simulink model "MagnetotorquersDynamics_part2"  (R2012b)
settings: Solver=ode1  StartTime=0.0  StopTime=2000  FixedStep=0.1  RelTol=1e-3
InitFcn:
  | clear all;close all;clc;warning off all;
  | 
  | a=1/sqrt(3);
  | 
  | Z=[-a a a -a; -a -a a a; a a a a];
  | 
  | pinvZ=pinv(Z);
  | 
  | 
  | % Simulation run parameters
  | Rate=34.3; DeltaT=1/Rate;
  | 
  | % Maneuver Parameters
  | roll=0; pitch=0; yaw=30; roll=roll*pi/180; pitch=pitch*pi/180; yaw=yaw*pi/180;
  | SlewTime=5; SACengage=0;
  | Re=6371.2e3;mu=398601.2e9; %earth radius and universal gravitation constant
  | 
  | %Spacecraft orbit
  | h=180e3; %orbit altitude in meters
  | R=Re+h; %orbit radius from center of earth
  | we=0.000072921158553; %earth's angular velocity rad/solar sec(Vallado)
  | wo=sqrt(mu/(Re+h)^3);
  | 
  | 
  | %Spacecraft Inertia conditions
  | Ix=119.1259; Iy=150.6615; Iz=106.0288;
  | Ixy=0; Iyz=0; Ixz=0;
  | Imo=[Ix Ixy Ixz;
  | Ixy Iy Iyz;
  | Ixz Iyz Iz]; %Moment of inertia matrix
  | Iinv=inv(Imo); %Moment of inertia inverse goes in dynamics block
  | 
  | %Spacecraft initial Euler state angles and rates
  | phio=4*pi/180;thetao=-4*pi/180;psio=4*pi/180; %Initial Euler Angles
  | phidoto=0.15*pi/180;thetadoto=0.15*pi/180;psidoto=0.15*pi/180; %Initial Euler Rates
  | alfinit=[phio thetao psio];
  | winit=[phidoto thetadoto psidoto];
  | 
  | %Calculation of initial quaternion (qo) and angular momentum (Ho)
  | s1=sin(phio/2);s2=sin(thetao/2);s3=sin(psio/2);c1=cos(phio/2);c2=cos(thetao/2);c3=cos(psio/2);
  | q1o=s1*c2*c3-c1*s2*s3;
  | q2o=c1*s2*c3+s1*c2*s3; %Wie pg. 321
  | q3o=c1*c2*s3-s1*s2*c3;
  | q4o=c1*c2*c3+s1*s2*s3;
  | S1=sin(phio);S2=sin(thetao);S3=sin(psio);C1=cos(phio);C2=cos(thetao);C3=cos(psio);
  | wxo=phidoto-psidoto*S2-wo*S3*C2;
  | wyo=thetadoto*C1+psidoto*C2*S1-wo*(C3*C1+S3*S2*S1);
  | wzo=psidoto*C2*C1-thetadoto*S1-wo*(S3*S2*C1-C3*S1);
  | qo=[q1o q2o q3o q4o];
  | Ho=Imo*[wxo wyo wzo]';
  | 
  | x=[4 4 4 2 2 2];%xmax
  | u=[2.1 2.1 2.1];%umax
  | J=[Ix Iy Iz];  % J of the system
  | 
  | Jinv=J';
  | 
  | hom=0.001; %rad/s
  | N=0;
  | %Linear quadratic Regulator
  | A=[0,0,0,1,0,0;0,0,0,0,1,0;0,0,0,0,0,1;4*((J(3)-J(2))/J(1))*(hom^2),0,0,0,0,((J(3)+J(1)-J(2))/J(1))*hom;0,3*((J(3)-J(1))/J(2))*(hom^2),0,0,0,0;0,0,((J(1)-J(2))/J(3))*(hom^2),(((J(2)-J(1)-J(3))/J(3))*hom),0,0];
  | B=[0,0,0;0,0,0;0,0,0;1/J(1),0,0;0,1/J(2),0;0,0,1/J(3)];
  | Q=[1/(x(1)^2),0,0,0,0,0;0,1/(x(2)^2),0,0,0,0;0,0,1/(x(3)^2),0,0,0;0,0,0,1/(x(4)^2),0,0;0,0,0,0,1/(x(5)^2),0;0,0,0,0,0,1/(x(6)^2)];
  | R=[100/(u(1)^2),0,0;0,100/(u(2)^2),0;0,0,100/(u(3)^2)];
  | 
  |  K=lqr(A,B,Q,R,N);
  | 
  | %State Estimator
  | 
  | %C=[1,0,0,0,0,0;0,1,0,0,0,0;0,0,1,0,0,0;0,0,0,0,0,0;0,0,0,0,0,0;0,0,0,0,0,0];
  | 
  | C=eye(6,6);
  | Q1=eye(6,6);
  | R1=eye(6,6);
  | 
  | L=[lqr(A',C',Q1,R1)]';
  | 
  | %Magnetic Field
  | 
  | Bxe=22791*10^(-9);% nT
  | Bye=0;
  | Bze=-11452*10^(-9);
  | 
  | Bx=22.791;% nT
  | By=0;
  | Bz=-11.452;
  | 
  | Be=[Bxe Bye Bze];
  | 
  | Bi=[Bx By Bz];
  | 
  | B=[0 Bz -By; -Bz 0 Bx; By -Bx 0];
  | 
  | Intialrate=[1.8*pi/180;1.8*pi/180;1.8*pi/180];
  | 
  | %Intialrate=[1.8*pi/180;0;1.8*pi/180];
  | %Intialrate=[0.8*pi/180;0.8*pi/180;0.8*pi/180];
  | 
  | BoB=1;
libraries: aerospace x7
settings Model: Creator=bleonard  LastModifiedBy=Grompone
settings DataIOCC: SignalLoggingSaveFormat=ModelDataLogs
settings OptimizationCC: InitFltsAndDblsToZero=on
settings DebuggingCC: SaveWithParameterizedLinksMsg=none  MultiTaskCondExecSysMsg=none  FcnCallInpInsideContextMsg=EnableAllAsWarning  StrictBusMsg=None
settings RTWCC: IncludeERTFirstTime=on
settings GRTTargetCC: CombineOutputUpdateFcns=off  GRTInterface=on

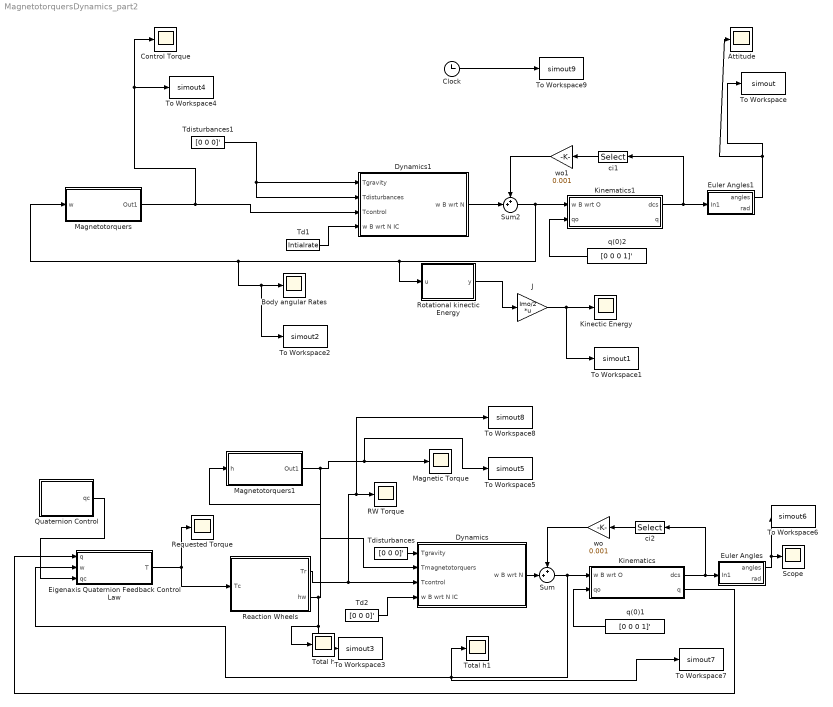
== system MagnetotorquersDynamics_part2 ==
  Attitude : Scope
      settings: YMin=-200  YMax=200  SaveName=ScopeData2
  Body angular Rates : Scope
      settings: YMin=-0.04  YMax=0.05  SaveName=ScopeData7
  Clock : Clock
  Control Torque : Scope
      settings: YMin=-1e-06  YMax=1.75e-06  SaveName=ScopeData5
  Dynamics : Subsystem
  Dynamics1 : Subsystem
  Eigenaxis Quaternion Feedback Control Law : Subsystem
  Euler Angles : Subsystem
  Euler Angles1 : Subsystem
  J : Gain  Gain=Imo/2  Multiplication=Matrix(K*u)  SaturateOnIntegerOverflow=on  OutDataTypeStr=Inherit: Same as input  ParamDataTypeStr=Inherit: Same as input
  Kinectic Energy : Scope
      settings: ShowLegends=on  YMin=-200  YMax=200  SaveName=ScopeData12
  Kinematics : Subsystem
  Kinematics1 : Subsystem
  Magnetic Torque : Scope
      settings: YMin=-7e-09  YMax=8e-09  SaveName=ScopeData15
  Magnetotorquers : Subsystem
  Magnetotorquers1 : Subsystem
  Quaternion Control : MATLAB Function  TreatAsAtomicUnit=on
  RW Torque : Scope
      settings: SaveName=ScopeData10
  Reaction Wheels : Subsystem
  Requested Torque : Scope
  Rotational kinectic Energy : MATLAB Function  TreatAsAtomicUnit=on
  Scope : Scope
      settings: YMin=-200  YMax=200
  Sum : Sum  Inputs=++|
  Sum2 : Sum  Inputs=++|
  Td1 : Constant  Value=Intialrate
  Td2 : Constant  Value=[0 0 0]'
  Tdisturbances : Constant  Value=[0 0 0]'
  Tdisturbances1 : Constant  Value=[0 0 0]'
  To Workspace : ToWorkspace  VariableName=simout  SampleTime=-1  SaveFormat=Timeseries
  To Workspace1 : ToWorkspace  VariableName=simout1  SampleTime=-1  SaveFormat=Timeseries
  To Workspace2 : ToWorkspace  VariableName=simout2  SampleTime=-1  SaveFormat=Timeseries
  To Workspace3 : ToWorkspace  VariableName=simout3  SampleTime=-1  SaveFormat=Timeseries
  To Workspace4 : ToWorkspace  VariableName=simout4  SampleTime=-1  SaveFormat=Timeseries
  To Workspace5 : ToWorkspace  VariableName=simout5  SampleTime=-1  SaveFormat=Timeseries
  To Workspace6 : ToWorkspace  VariableName=simout6  SampleTime=-1  SaveFormat=Timeseries
  To Workspace7 : ToWorkspace  VariableName=simout7  SampleTime=-1  SaveFormat=Timeseries
  To Workspace8 : ToWorkspace  VariableName=simout8  SampleTime=-1  SaveFormat=Timeseries
  To Workspace9 : ToWorkspace  VariableName=simout9  SampleTime=-1  SaveFormat=Timeseries
  Total h : Scope
      settings: YMin=-7e-09  YMax=8e-09  SaveName=ScopeData16
  Total h1 : Scope
      settings: YMin=-7e-09  YMax=8e-09  SaveName=ScopeData3
  ci1 : Selector  InputPortWidth=9  IndexOptions=Index vector (dialog)  Indices=[4 5 6]  OutputSizes=1
  ci2 : Selector  InputPortWidth=9  IndexOptions=Index vector (dialog)  Indices=[4 5 6]  OutputSizes=1
  q(0)1 : Constant  Value=[0 0 0 1]'
  q(0)2 : Constant  Value=[0 0 0 1]'
  wo : Gain  Gain=0.001
  wo1 : Gain  Gain=0.001
  wires:
  Sum/1 -> Total h1/1, To Workspace7/1, Eigenaxis Quaternion Feedback Control Law/2(w), Kinematics/1(w B wrt O)
  Kinematics/1(dcs) -> ci2/1, Euler Angles/1(In1)
  ci2/1 -> wo/1
  Euler Angles/1(angles) -> Scope/1, To Workspace6/1
  Kinematics/2(q) -> Eigenaxis Quaternion Feedback Control Law/1(q)
  Tdisturbances/1 -> Dynamics/1(Tgravity)
  Td2/1 -> Dynamics/4(w B wrt N IC)
  wo/1 -> Sum/1
  Eigenaxis Quaternion Feedback Control Law/1(T) -> Reaction Wheels/1(Tc), Requested Torque/1
  Reaction Wheels/1(Tr) -> To Workspace8/1, RW Torque/1, Dynamics/3(Tcontrol)
  Dynamics/1(w B wrt N) -> Sum/2
  q(0)1/1 -> Kinematics/2(qo)
  Quaternion Control/1(qc) -> Eigenaxis Quaternion Feedback Control Law/3(qc)
  Sum2/1 -> Rotational kinectic Energy/1(u), To Workspace2/1, Body angular Rates/1, Magnetotorquers/1(w), Kinematics1/1(w B wrt O)
  Kinematics1/1(dcs) -> ci1/1, Euler Angles1/1(In1)
  ci1/1 -> wo1/1
  Euler Angles1/1(angles) -> Attitude/1, To Workspace/1
  Tdisturbances1/1 -> Dynamics1/1(Tgravity), Dynamics1/2(Tdisturbances)
  Magnetotorquers/1(Out1) -> To Workspace4/1, Control Torque/1, Dynamics1/3(Tcontrol)
  Dynamics1/1(w B wrt N) -> Sum2/2
  q(0)2/1 -> Kinematics1/2(qo)
  Td1/1 -> Dynamics1/4(w B wrt N IC)
  wo1/1 -> Sum2/1
  Magnetotorquers1/1(Out1) -> Dynamics/2(Tmagnetotorquers), To Workspace5/1, Magnetic Torque/1
  Rotational kinectic Energy/1(y) -> J/1
  J/1 -> To Workspace1/1, Kinectic Energy/1
  Reaction Wheels/2(hw) -> Total h/1, To Workspace3/1, Magnetotorquers1/1(h)
  Clock/1 -> To Workspace9/1

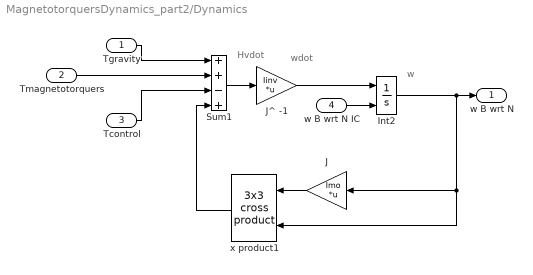
== system MagnetotorquersDynamics_part2/Dynamics ==
  note: wdot
  note: Hvdot
  note: w
  Tgravity : Inport
  Tmagnetotorquers : Inport  Port=2
  Tcontrol : Inport  Port=3
  w B wrt N IC : Inport  Port=4
  "   J^ -1" : Gain  Gain=Iinv  Multiplication=Matrix(K*u)  SaturateOnIntegerOverflow=on  OutDataTypeStr=Inherit: Same as input  ParamDataTypeStr=Inherit: Same as input
  Int2 : Integrator  InitialConditionSource=external  InitialCondition="[0  -0.001  0]'"
  J : Gain  Gain=Imo  Multiplication=Matrix(K*u)  SaturateOnIntegerOverflow=on  OutDataTypeStr=Inherit: Same as input  ParamDataTypeStr=Inherit: Same as input
  Sum1 : Sum  Inputs=++-+  SaturateOnIntegerOverflow=on  InputSameDT=on  OutDataTypeStr=Inherit: Same as first input
  x product1 : aerospace/Axes Transformations/3x3 cross product
  w B wrt N : Outport
  wires:
  Sum1/1 -> "   J^ -1"/1
  Int2/1 -> J/1, x product1/2, w B wrt N/1
  x product1/1 -> Sum1/4
  "   J^ -1"/1 -> Int2/1
  J/1 -> x product1/1
  Tgravity/1 -> Sum1/1
  Tmagnetotorquers/1 -> Sum1/2
  Tcontrol/1 -> Sum1/3
  w B wrt N IC/1 -> Int2/2

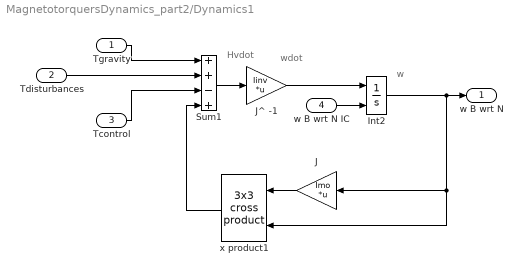
== system MagnetotorquersDynamics_part2/Dynamics1 ==
  note: wdot
  note: Hvdot
  note: w
  Tgravity : Inport
  Tdisturbances : Inport  Port=2
  Tcontrol : Inport  Port=3
  w B wrt N IC : Inport  Port=4
  "   J^ -1" : Gain  Gain=Iinv  Multiplication=Matrix(K*u)  SaturateOnIntegerOverflow=on  OutDataTypeStr=Inherit: Same as input  ParamDataTypeStr=Inherit: Same as input
  Int2 : Integrator  InitialConditionSource=external  InitialCondition="[0  -0.001  0]'"
  J : Gain  Gain=Imo  Multiplication=Matrix(K*u)  SaturateOnIntegerOverflow=on  OutDataTypeStr=Inherit: Same as input  ParamDataTypeStr=Inherit: Same as input
  Sum1 : Sum  Inputs=++-+  SaturateOnIntegerOverflow=on  InputSameDT=on  OutDataTypeStr=Inherit: Same as first input
  x product1 : aerospace/Axes Transformations/3x3 cross product
  w B wrt N : Outport
  wires:
  Sum1/1 -> "   J^ -1"/1
  Int2/1 -> J/1, x product1/2, w B wrt N/1
  x product1/1 -> Sum1/4
  "   J^ -1"/1 -> Int2/1
  J/1 -> x product1/1
  Tgravity/1 -> Sum1/1
  Tdisturbances/1 -> Sum1/2
  Tcontrol/1 -> Sum1/3
  w B wrt N IC/1 -> Int2/2

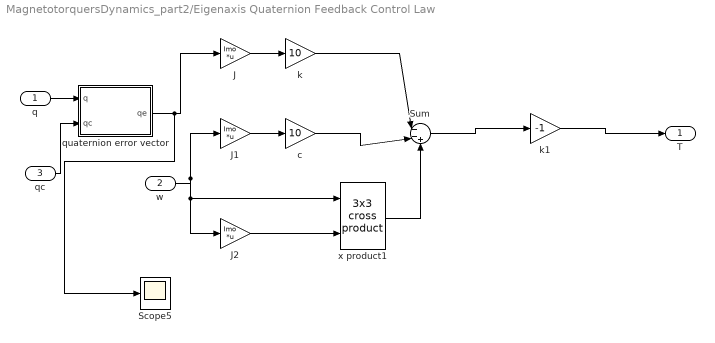
== system MagnetotorquersDynamics_part2/Eigenaxis Quaternion Feedback Control Law ==
  q : Inport
  w : Inport  Port=2
  qc : Inport  Port=3
  J : Gain  Gain=Imo  Multiplication=Matrix(K*u)
  J1 : Gain  Gain=Imo  Multiplication=Matrix(K*u)
  J2 : Gain  Gain=Imo  Multiplication=Matrix(K*u)
  Scope5 : Scope
      settings: YMin=-200  YMax=200  SaveName=ScopeData6
  Sum : Sum  Inputs=|--+
  c : Gain  Gain=10
  k : Gain  Gain=10
  k1 : Gain  Gain=-1
  quaternion error vector : MATLAB Function  TreatAsAtomicUnit=on
  x product1 : aerospace/Axes Transformations/3x3 cross product
  T : Outport
  wires:
  J/1 -> k/1
  quaternion error vector/1(qe) -> Scope5/1, J/1
  J1/1 -> c/1
  w/1 -> J1/1, x product1/1, J2/1
  k/1 -> Sum/1
  c/1 -> Sum/2
  x product1/1 -> Sum/3
  q/1 -> quaternion error vector/1(q)
  qc/1 -> quaternion error vector/2(qc)
  J2/1 -> x product1/2
  Sum/1 -> k1/1
  k1/1 -> T/1

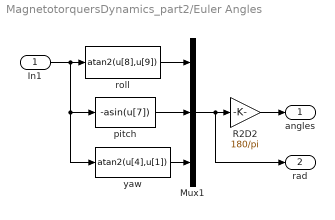
== system MagnetotorquersDynamics_part2/Euler Angles ==
  In1 : Inport
  Mux1 : Mux  Inputs=3
  R2D2 : Gain  Gain=180/pi  SampleTime=0.1
  pitch : Fcn  Expr=-asin(u[7])
  roll : Fcn  Expr=atan2(u[8],u[9])
  yaw : Fcn  Expr=atan2(u[4],u[1])
  angles : Outport
  rad : Outport  Port=2
  wires:
  roll/1 -> Mux1/1
  yaw/1 -> Mux1/3
  pitch/1 -> Mux1/2
  Mux1/1 -> rad/1, R2D2/1
  In1/1 -> roll/1, pitch/1, yaw/1
  R2D2/1 -> angles/1

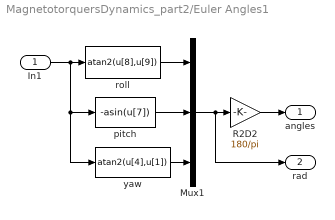
== system MagnetotorquersDynamics_part2/Euler Angles1 ==
  In1 : Inport
  Mux1 : Mux  Inputs=3
  R2D2 : Gain  Gain=180/pi  SampleTime=0.1
  pitch : Fcn  Expr=-asin(u[7])
  roll : Fcn  Expr=atan2(u[8],u[9])
  yaw : Fcn  Expr=atan2(u[4],u[1])
  angles : Outport
  rad : Outport  Port=2
  wires:
  roll/1 -> Mux1/1
  yaw/1 -> Mux1/3
  pitch/1 -> Mux1/2
  Mux1/1 -> rad/1, R2D2/1
  In1/1 -> roll/1, pitch/1, yaw/1
  R2D2/1 -> angles/1

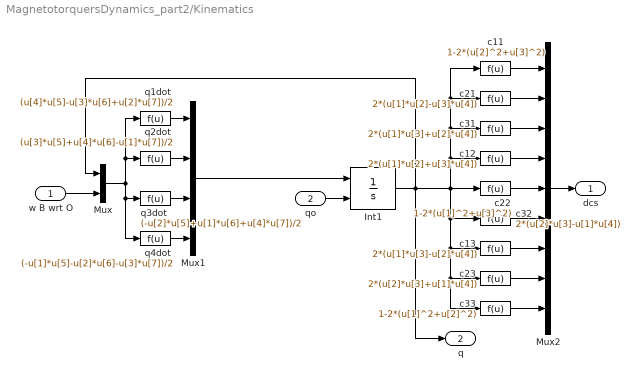
== system MagnetotorquersDynamics_part2/Kinematics ==
  w B wrt O : Inport
  qo : Inport  Port=2
  Int1 : Integrator  InitialConditionSource=external  InitialCondition=[0 0 -0.1]'
  Mux : Mux  Inputs=2
  Mux1 : Mux
  Mux2 : Mux  Inputs=9
  c11 : Fcn  Expr=1-2*(u[2]^2+u[3]^2)
  c12 : Fcn  Expr=2*(u[1]*u[2]+u[3]*u[4])
  c13 : Fcn  Expr=2*(u[1]*u[3]-u[2]*u[4])
  c21 : Fcn  Expr=2*(u[1]*u[2]-u[3]*u[4])
  c22 : Fcn  Expr=1-2*(u[1]^2+u[3]^2)
  c23 : Fcn  Expr=2*(u[2]*u[3]+u[1]*u[4])
  c31 : Fcn  Expr=2*(u[1]*u[3]+u[2]*u[4])
  c32 : Fcn  Expr=2*(u[2]*u[3]-u[1]*u[4])
  c33 : Fcn  Expr=1-2*(u[1]^2+u[2]^2)
  q1dot : Fcn  Expr=(u[4]*u[5]-u[3]*u[6]+u[2]*u[7])/2
  q2dot : Fcn  Expr=(u[3]*u[5]+u[4]*u[6]-u[1]*u[7])/2
  q3dot : Fcn  Expr=(-u[2]*u[5]+u[1]*u[6]+u[4]*u[7])/2
  q4dot : Fcn  Expr=(-u[1]*u[5]-u[2]*u[6]-u[3]*u[7])/2
  dcs : Outport
  q : Outport  Port=2
  wires:
  Mux/1 -> q4dot/1, q3dot/1, q1dot/1, q2dot/1
  q1dot/1 -> Mux1/1
  q2dot/1 -> Mux1/2
  q3dot/1 -> Mux1/3
  q4dot/1 -> Mux1/4
  Int1/1 -> Mux/1, c22/1, c11/1, c21/1, c31/1, c12/1, c32/1, c13/1, c33/1, c23/1, q/1
  c11/1 -> Mux2/1
  c22/1 -> Mux2/5
  c33/1 -> Mux2/9
  c21/1 -> Mux2/2
  c31/1 -> Mux2/3
  c12/1 -> Mux2/4
  c32/1 -> Mux2/6
  c13/1 -> Mux2/7
  c23/1 -> Mux2/8
  Mux1/1 -> Int1/1
  w B wrt O/1 -> Mux/2
  Mux2/1 -> dcs/1
  qo/1 -> Int1/2

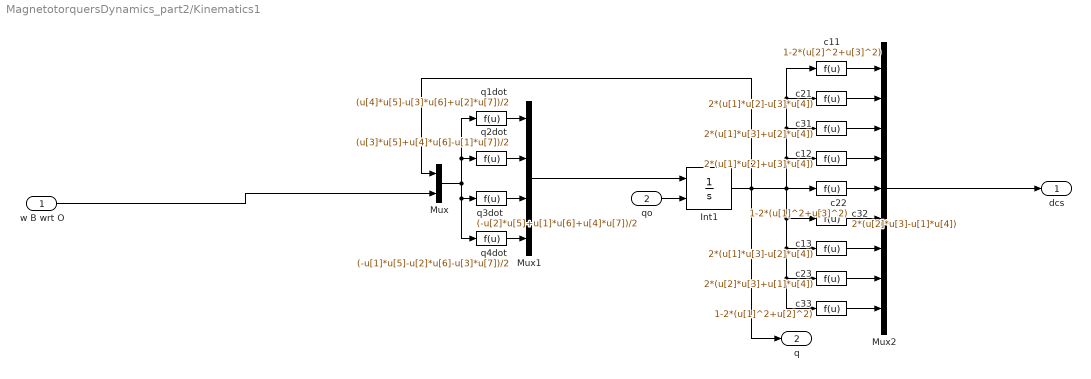
== system MagnetotorquersDynamics_part2/Kinematics1 ==
  w B wrt O : Inport
  qo : Inport  Port=2
  Int1 : Integrator  InitialConditionSource=external  InitialCondition=[0 0 -0.1]'
  Mux : Mux  Inputs=2
  Mux1 : Mux
  Mux2 : Mux  Inputs=9
  c11 : Fcn  Expr=1-2*(u[2]^2+u[3]^2)
  c12 : Fcn  Expr=2*(u[1]*u[2]+u[3]*u[4])
  c13 : Fcn  Expr=2*(u[1]*u[3]-u[2]*u[4])
  c21 : Fcn  Expr=2*(u[1]*u[2]-u[3]*u[4])
  c22 : Fcn  Expr=1-2*(u[1]^2+u[3]^2)
  c23 : Fcn  Expr=2*(u[2]*u[3]+u[1]*u[4])
  c31 : Fcn  Expr=2*(u[1]*u[3]+u[2]*u[4])
  c32 : Fcn  Expr=2*(u[2]*u[3]-u[1]*u[4])
  c33 : Fcn  Expr=1-2*(u[1]^2+u[2]^2)
  q1dot : Fcn  Expr=(u[4]*u[5]-u[3]*u[6]+u[2]*u[7])/2
  q2dot : Fcn  Expr=(u[3]*u[5]+u[4]*u[6]-u[1]*u[7])/2
  q3dot : Fcn  Expr=(-u[2]*u[5]+u[1]*u[6]+u[4]*u[7])/2
  q4dot : Fcn  Expr=(-u[1]*u[5]-u[2]*u[6]-u[3]*u[7])/2
  dcs : Outport
  q : Outport  Port=2
  wires:
  Mux/1 -> q4dot/1, q3dot/1, q1dot/1, q2dot/1
  q1dot/1 -> Mux1/1
  q2dot/1 -> Mux1/2
  q3dot/1 -> Mux1/3
  q4dot/1 -> Mux1/4
  Int1/1 -> Mux/1, c22/1, c11/1, c21/1, c31/1, c12/1, c32/1, c13/1, c33/1, c23/1, q/1
  c11/1 -> Mux2/1
  c22/1 -> Mux2/5
  c33/1 -> Mux2/9
  c21/1 -> Mux2/2
  c31/1 -> Mux2/3
  c12/1 -> Mux2/4
  c32/1 -> Mux2/6
  c13/1 -> Mux2/7
  c23/1 -> Mux2/8
  Mux1/1 -> Int1/1
  qo/1 -> Int1/2
  w B wrt O/1 -> Mux/2
  Mux2/1 -> dcs/1

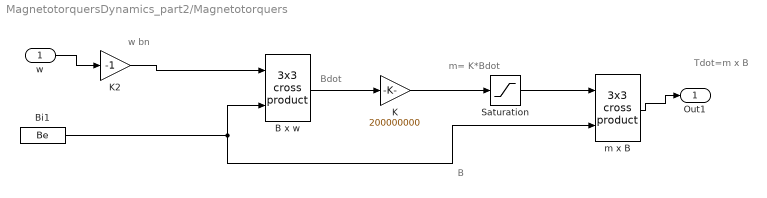
== system MagnetotorquersDynamics_part2/Magnetotorquers ==
  note: w bn
  note: B
  note: m= K*Bdot
  note: Tdot=m x B
  note: Bdot
  w : Inport
  B x w : aerospace/Axes Transformations/3x3 cross product
  Bi1 : Constant  Value=Be
  K : Gain  Gain=200000000
  K2 : Gain  Gain=-1
  Saturation : Saturate  UpperLimit=110  LowerLimit=-110
  m x B : aerospace/Axes Transformations/3x3 cross product
  Out1 : Outport
  wires:
  B x w/1 -> K/1
  m x B/1 -> Out1/1
  K/1 -> Saturation/1
  w/1 -> K2/1
  Bi1/1 -> m x B/2, B x w/2
  K2/1 -> B x w/1
  Saturation/1 -> m x B/1

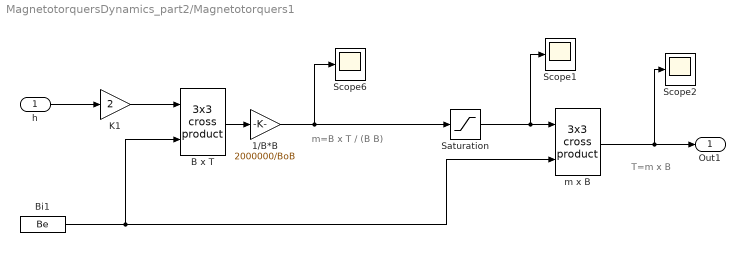
== system MagnetotorquersDynamics_part2/Magnetotorquers1 ==
  note: m=B x T / (B B)
  note: T=m x B
  h : Inport
  1/B*B : Gain  Gain=2000000/BoB
  B x T : aerospace/Axes Transformations/3x3 cross product
  Bi1 : Constant  Value=Be
  K1 : Gain  Gain=2
  Saturation : Saturate  UpperLimit=110  LowerLimit=-110
  Scope1 : Scope
      settings: YMin=-6.5  YMax=0.5  SaveName=ScopeData9
  Scope2 : Scope
      settings: YMin=-0.000225  YMax=0.00035  SaveName=ScopeData11
  Scope6 : Scope
      settings: YMin=-0.00225  YMax=0.002  SaveName=ScopeData8
  m x B : aerospace/Axes Transformations/3x3 cross product
  Out1 : Outport
  wires:
  m x B/1 -> Scope2/1, Out1/1
  Saturation/1 -> Scope1/1, m x B/1
  h/1 -> K1/1
  K1/1 -> B x T/1
  Bi1/1 -> m x B/2, B x T/2
  B x T/1 -> 1/B*B/1
  1/B*B/1 -> Scope6/1, Saturation/1

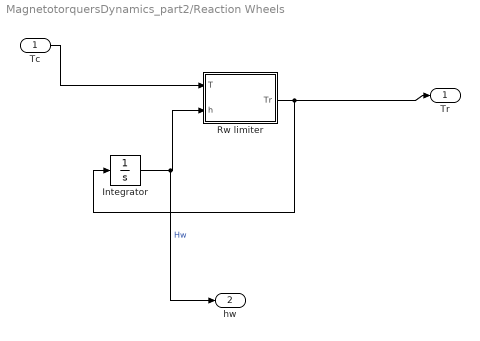
== system MagnetotorquersDynamics_part2/Reaction Wheels ==
  Tc : Inport
  Integrator : Integrator  InitialCondition=[0 0 0]
  Rw limiter : MATLAB Function  TreatAsAtomicUnit=on
  Tr : Outport
  hw : Outport  Port=2
  wires:
  Integrator/1 -> hw/1, Rw limiter/2(h)  "Hw"
  Rw limiter/1(Tr) -> Integrator/1, Tr/1
  Tc/1 -> Rw limiter/1(T)

== matlab function MagnetotorquersDynamics_part2/Quaternion Control ==
  data: qc output
function qc = fcn
%#codegen

alfa=120*pi/180;

e1=1/sqrt(3);
e2=1/sqrt(3);
e3=1/sqrt(3);


q1=sin(alfa/2)*e1;
q2=sin(alfa/2)*e2;
q3=sin(alfa/2)*e3;
q4=cos(alfa/2);


qc = [q1 q2 q3 q4];

== matlab function MagnetotorquersDynamics_part2/Reaction Wheels/Rw limiter ==
  data: T input; Tr output; h input
function Tr = fcn(T,h)
%#eml



hmax=20; %absolute maximum momentum RW

Tmax=0.1; %absolute maximum Torque RW

Trc=zeros(3,1);
Tr=zeros(3,1);

if abs(h(1))<hmax

if abs(T(1))>Tmax
    
    Trc(1)=Tmax;
    
else
    
    Trc(1)=abs(T(1));
    
end

else
    
  Trc(1)=0;
  
end

Tr(1)=sign(T(1))*Trc(1);

if abs(h(2))<hmax

if abs(T(2))>Tmax
    
    Trc(2)=Tmax;
    
else
    
    Trc(2)=abs(T(2));
    
end

else
    
  Trc(2)=0;
  
end

Tr(2)=sign(T(2))*Trc(2);

if abs(h(3))<hmax

if abs(T(3))>Tmax
    
    Trc(3)=Tmax;
    
else
    
    Trc(3)=abs(T(3));
    
end

else
    
  Trc(3)=0;
  
end

Tr(3)=sign(T(3))*Trc(3);

== matlab function MagnetotorquersDynamics_part2/Eigenaxis Quaternion Feedback Control Law/quaternion error vector ==
  data: q input; qe output; qc input
function qe = fcn(q,qc)
%#codegen

qcm=[qc(4) qc(3) -qc(2) -qc(1);-qc(3) qc(4) qc(1) -qc(2);qc(2) -qc(1) qc(4) -qc(3);qc(1) qc(2) qc(3) qc(4)];


qem = qcm*q; 

qe=[qem(1) qem(2) qem(3)]';

== matlab function MagnetotorquersDynamics_part2/Rotational kinectic Energy ==
  data: u input; y output
function y = fcn(u)
%#codegen
us=zeros(3,1);
us(1)=u(1)^2;
us(2)=u(2)^2;
us(3)=u(3)^2;

y=zeros(3,1);

y = us;
